simulink model "HeartModelECGPrint"  (R2014a)
settings: Solver=FixedStepDiscrete  StartTime=0.0  StopTime=100  FixedStep=0.01  RelTol=1e-3
values from neighbouring files (symbols this model uses):
  Atr_refrD = 50    [matlab.mat]
  AV_alpha = 150    [matlab.mat]
  AV_anteDMin = 100    [matlab.mat]
  AV_beta = 250    [matlab.mat]
  AV_delta = 10    [matlab.mat]
  AV_k4 = 0.03    [matlab.mat]
  AV_refrDMin = 50    [matlab.mat]
  AV_retroDMin = 100    [matlab.mat]
  AV_tauC = 100    [matlab.mat]
  AV_theta = 10    [matlab.mat]
  AV_tr = 500    [matlab.mat]
  AV_Vr = -90    [matlab.mat]
  AV_Vt = -40    [matlab.mat]
  PM_TAVI = 150    [matlab.mat]
  PM_TLRI = 1000    [matlab.mat]
  PM_TPVAB = 50    [matlab.mat]
  PM_TPVARP = 250    [matlab.mat]
  PM_TURI = 400    [matlab.mat]
  PM_TVRP = 320    [matlab.mat]
  RA_anteD = 75.8904109589    [matlab.mat]
  RA_retroD = 30    [matlab.mat]
  RV_anteD = 50    [matlab.mat]
  RV_retroD = 50    [matlab.mat]
  SA_d = 880.219178082    [matlab.mat]
  SA_dV = 50    [matlab.mat]
  SA_ectopD = 10400    [matlab.mat]
  SA_ectopdV = 50    [matlab.mat]
  SA_noiseD = 1000000    [matlab.mat]
  VRG_d = 3000    [matlab.mat]
  VRG_ectopD = 30450    [matlab.mat]
  VRG_noiseD = 1000000    [matlab.mat]
  Vtr_refrD = 252.054794521    [matlab.mat]
libraries: simulink x4
settings Model: Creator=alexandru  LastModifiedBy=barbot
settings DataIOCC: LimitDataPoints=off  SaveOutput=off  SignalLogging=off  DSMLogging=off  SaveTime=off
settings HardwareCC: TargetBitPerLong=64  TargetBitPerPointer=64  TargetLongLongMode=on  TargetIntDivRoundTo=Zero  TargetEndianess=LittleEndian  TargetWordSize=64  TargetHWDeviceType=MATLAB Host  ProdEqTarget=off
settings RTWCC: SystemTargetFile=rsim.tlc  GenCodeOnly=on  PackageGeneratedCodeAndArtifacts=on  PackageName=idhp_model_heart_realtime  TemplateMakefile=rsim_default_tmf  Description=Rapid Simulation Target  ProcessScript=rsim_make_rtw_hook
settings RSimTargetCC: ERTMultiwordTypeDef=System defined  ERTMultiwordLength=256  EnableShiftOperators=on

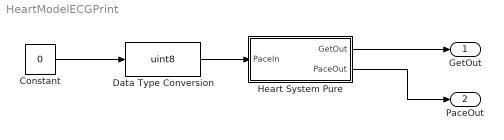
== system HeartModelECGPrint ==
  Constant : Constant  Value=0
  Data Type Conversion : DataTypeConversion  OutDataTypeStr=uint8
  Heart System Pure : Subsystem
  GetOut : Outport
  PaceOut : Outport  Port=2
  wires:
  Data Type Conversion/1 -> Heart System Pure/1(PaceIn)
  Heart System Pure/1(GetOut) -> GetOut/1
  Heart System Pure/2(PaceOut) -> PaceOut/1
  Constant/1 -> Data Type Conversion/1

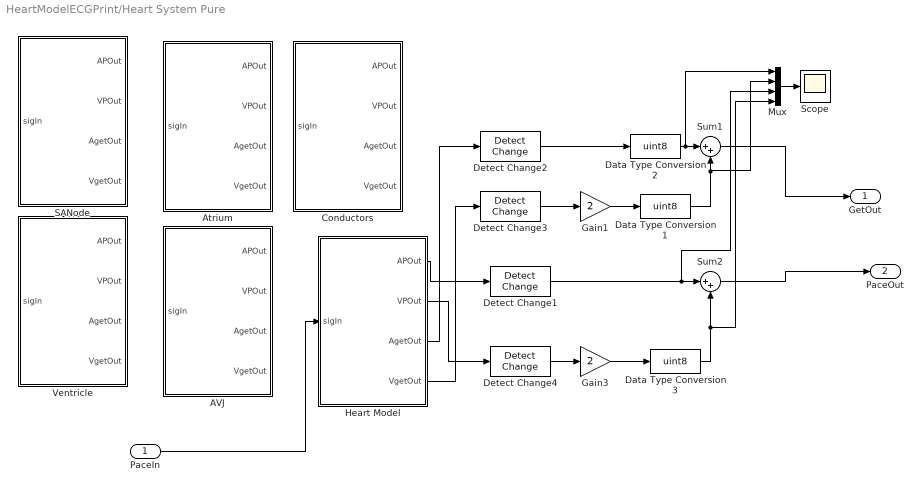
== system HeartModelECGPrint/Heart System Pure ==
  PaceIn : Inport
  AVJ : Stateflow chart  Priority=1  TreatAsAtomicUnit=on
  Atrium : Stateflow chart  Priority=1  TreatAsAtomicUnit=on
  Conductors : Stateflow chart  Priority=1  TreatAsAtomicUnit=on
  Data Type Conversion1 : DataTypeConversion  OutDataTypeStr=uint8
  Data Type Conversion2 : DataTypeConversion  OutDataTypeStr=uint8
  Data Type Conversion3 : DataTypeConversion  OutDataTypeStr=uint8
  Detect Change{1..4} (4 alike) : simulink/Logic and Bit Operations/Detect Change  vinit=0  InputProcessing=Inherited  OutDataTypeStr=uint8
  Gain1 : Gain  Gain=2
  Gain3 : Gain  Gain=2
  Heart Model : Stateflow chart  Priority=1  TreatAsAtomicUnit=on
  Mux : Mux
  SANode : Stateflow chart  Priority=1  TreatAsAtomicUnit=on
  Scope : Scope
  Sum1 : Sum  Inputs=|++
  Sum2 : Sum  Inputs=|++
  Ventricle : Stateflow chart  Priority=1  TreatAsAtomicUnit=on
  GetOut : Outport
  PaceOut : Outport  Port=2
  wires:
  Detect Change3/1 -> Gain1/1
  Gain1/1 -> Data Type Conversion1/1
  Sum1/1 -> GetOut/1
  Data Type Conversion1/1 -> Mux/2, Sum1/2
  Detect Change2/1 -> Data Type Conversion2/1
  Data Type Conversion2/1 -> Mux/1, Sum1/1
  Heart Model/1(APOut) -> Detect Change1/1
  Heart Model/2(VPOut) -> Detect Change4/1
  Detect Change4/1 -> Gain3/1
  Gain3/1 -> Data Type Conversion3/1
  Data Type Conversion3/1 -> Mux/4, Sum2/2
  Detect Change1/1 -> Mux/3, Sum2/1
  Sum2/1 -> PaceOut/1
  PaceIn/1 -> Heart Model/1(sigIn)
  Heart Model/4(VgetOut) -> Detect Change3/1
  Heart Model/3(AgetOut) -> Detect Change2/1
  Mux/1 -> Scope/1

== stateflow chart HeartModelECGPrint/Heart System Pure/SANode ==
  state SANodeEctopic
    state q0
    q0 -> q0 : after(SA_ectopD),
        | !Abeat , {a_dV=SA_ectopdV}
    (default) -> q0
  state SANode
    state Wait4ABeat
    state Wait4ASynch
    Wait4ABeat -> Wait4ASynch [order 2] : after(SA_d),!Abeat,
        | {a_dV=SA_dV}
    (default) -> Wait4ABeat
    Wait4ASynch -> Wait4ABeat : ?NextAtrBeat
    Wait4ABeat -> Wait4ABeat [order 1] : ?NextAtrBeat
  data: Atr_refrD parameter; AV_alpha parameter; AV_anteDMin parameter; AV_beta parameter; AV_delta parameter; AV_k4 parameter; AV_refrDMin parameter; AV_retroDMin parameter; AV_tauC parameter; AV_theta parameter; AV_tr parameter; AV_Vr parameter; AV_Vt parameter; RA_anteD parameter; RA_retroD parameter; RV_anteD parameter; RV_retroD parameter; SA_d parameter; SA_dV parameter; SA_ectopD parameter; SA_ectopdV parameter; SA_noiseD parameter; VRG_d parameter; VRG_ectopD parameter; VRG_noiseD parameter; Vtr_refrD parameter; a_dV local double; avj_tRec local double; sigIn input uint8; clk local double; PM_TAVI parameter; PM_TLRI parameter; PM_TPVAB parameter; PM_TPVARP parameter; PM_TURI parameter; PM_TVRP parameter; data local double
  events: Abeat local FUNCTION_CALL_EVENT; AtrRetroReached local FUNCTION_CALL_EVENT; arg local FUNCTION_CALL_EVENT; retroAVJ local FUNCTION_CALL_EVENT; AVJAnteReached local FUNCTION_CALL_EVENT; NextAtrBeat local FUNCTION_CALL_EVENT; AVJRetroReached local FUNCTION_CALL_EVENT; anteAVJ local FUNCTION_CALL_EVENT; vrg local FUNCTION_CALL_EVENT; VtrAnteReached local FUNCTION_CALL_EVENT; AVJRetroExit local FUNCTION_CALL_EVENT; AVJAnteExit local FUNCTION_CALL_EVENT; NextVtrBeat local FUNCTION_CALL_EVENT; Vbeat local FUNCTION_CALL_EVENT; AP local EITHER_EDGE_EVENT; VP local EITHER_EDGE_EVENT; APOut output EITHER_EDGE_EVENT; VPOut output EITHER_EDGE_EVENT; AS local RISING_EDGE_EVENT; VS local RISING_EDGE_EVENT; Aget local EITHER_EDGE_EVENT; Vget local EITHER_EDGE_EVENT; Aintrinsic local EITHER_EDGE_EVENT; Anoise local EITHER_EDGE_EVENT; Aretro local EITHER_EDGE_EVENT; Vintrinsic local EITHER_EDGE_EVENT; Vnoise local EITHER_EDGE_EVENT; Vante local EITHER_EDGE_EVENT; AgetOut output EITHER_EDGE_EVENT; VgetOut output EITHER_EDGE_EVENT; APElectr local RISING_EDGE_EVENT; VPElectr local EITHER_EDGE_EVENT

== stateflow chart HeartModelECGPrint/Heart System Pure/Heart Model ==
  state Heart
    state SANodeEctopic [parallel]
      settings: executionOrder=10
      state q0
      Heart.SANodeEctopic.q0 -> Heart.SANodeEctopic.q0 : after(SA_ectopD),
          | !Abeat , {a_dV=SA_ectopdV}
      (default) -> Heart.SANodeEctopic.q0
    state RAConductor [parallel]
      settings: executionOrder=3
      state Ante
      state Empty
      state Retro
      Heart.RAConductor.Empty -> Heart.RAConductor.Ante [order 1] : ?arg
      Heart.RAConductor.Ante -> Heart.RAConductor.Empty [order 1] : ?retroAVJ
      (default) -> Heart.RAConductor.Empty
      Heart.RAConductor.Ante -> Heart.RAConductor.Empty [order 2] : after(RA_anteD),
          | !AVJAnteReached
      Heart.RAConductor.Empty -> Heart.RAConductor.Retro [order 2] : ?retroAVJ
      Heart.RAConductor.Retro -> Heart.RAConductor.Empty [order 1] : ?arg
      Heart.RAConductor.Retro -> Heart.RAConductor.Empty [order 2] : after(RA_retroD),
          | !AtrRetroReached
    state AVJOut [parallel]
      settings: executionOrder=1
      state Empty
      state Ante
      state Retro
      Heart.AVJOut.Ante -> Heart.AVJOut.Empty : after(AV_anteDMin+AV_alpha*exp(-avj_tRec/AV_tauC)),
          | !anteAVJ
      (default) -> Heart.AVJOut.Empty
      Heart.AVJOut.Empty -> Heart.AVJOut.Ante [order 1] : ?AVJAnteExit
      Heart.AVJOut.Retro -> Heart.AVJOut.Empty : after(AV_retroDMin+AV_alpha*exp(-avj_tRec/AV_tauC)),
          | !retroAVJ
      Heart.AVJOut.Empty -> Heart.AVJOut.Retro [order 2] : ?AVJRetroExit
    state RVConductor [parallel]
      settings: executionOrder=2
      state Empty
      state Ante
      state Retro
      (default) -> Heart.RVConductor.Empty
      Heart.RVConductor.Empty -> Heart.RVConductor.Ante [order 1] : ?anteAVJ
      Heart.RVConductor.Ante -> Heart.RVConductor.Empty [order 1] : ?vrg
      Heart.RVConductor.Ante -> Heart.RVConductor.Empty [order 2] : after(RV_anteD),
          | !VtrAnteReached
      Heart.RVConductor.Empty -> Heart.RVConductor.Retro [order 2] : ?vrg
      Heart.RVConductor.Retro -> Heart.RVConductor.Empty [order 1] : ?anteAVJ
      Heart.RVConductor.Retro -> Heart.RVConductor.Empty [order 2] : after(RV_retroD),
          | !AVJRetroReached
    state VRGEctopic [parallel]
      settings: executionOrder=8
      state q0
      (default) -> Heart.VRGEctopic.q0
      Heart.VRGEctopic.q0 -> Heart.VRGEctopic.q0 : after(VRG_ectopD), !Vbeat
    state VRG [parallel]
      settings: executionOrder=9
      state Wait4VBeat
      state Wait4VSynch
      (default) -> Wait4VBeat
      Wait4VBeat -> Wait4VSynch [order 2] : after(VRG_d), !Vbeat
      Wait4VSynch -> Wait4VBeat : ?NextVtrBeat
      Wait4VBeat -> Wait4VBeat [order 1] : ?NextVtrBeat
    state SANode [parallel]
      settings: executionOrder=4
      state Wait4ABeat
      state Wait4ASynch
      Wait4ABeat -> Wait4ASynch [order 2] : after(SA_d),!Abeat,
          | {a_dV=SA_dV}
      (default) -> Wait4ABeat
      Wait4ASynch -> Wait4ABeat : ?NextAtrBeat
      Wait4ABeat -> Wait4ABeat [order 1] : ?NextAtrBeat
    state AVJ [parallel]
      settings: executionOrder=7
      state Recovery
      state Ante
      state Refractory
      state Retro
      (default) -> Recovery : {avj_t4=timeToDep(AV_Vr);
          | ctime=0;
          | recoverylast=0;
          | antelast=0;
          | refractorylast=0;}
      Heart.AVJ.Ante -> Heart.AVJ.Refractory : after(avj_t4), !AVJAnteExit, {
          | avj_tRec=avj_tRec+(ctime-antelast);
          | avj_refr_0=initRefrPeriod(avj_tRec);
          | avj_refr=avj_refr_0;
          | refractorylast=ctime;}
      Recovery -> Heart.AVJ.Ante [order 1] : ?AVJAnteReached,{
          | avj_t4 = timeToDep(AV_Vr+ ...
          | (ctime-recoverylast)*AV_k4 + a_dV);
          | avj_tRec=ctime-recoverylast;
          | antelast=ctime;}
      Recovery -> Heart.AVJ.Refractory [order 2] : after(avj_t4), {
          | avj_tRec=avj_t4;
          | avj_refr_0=initRefrPeriod(avj_tRec);
          | avj_refr=avj_refr_0;
          | refractorylast=ctime;}
      Heart.AVJ.Refractory -> Heart.AVJ.Refractory [order 1] : ?AVJAnteReached,{
          | avj_refr=avj_refr-(ctime - refractorylast)+...
          | modulateRefrAnte((ctime - refractorylast),...
          | avj_refr_0,a_dV);
          | refractorylast=ctime;}
      Heart.AVJ.Refractory -> Recovery [order 3] : after(avj_refr), {
          | avj_t4=timeToDep(AV_Vr);
          | recoverylast=ctime;}
      Recovery -> Heart.AVJ.Retro [order 3] : ?AVJRetroReached,{
          | avj_tRec=ctime-recoverylast;
          | avj_refr_0=initRefrPeriod(avj_tRec);
          | avj_refr=avj_refr_0;}
      Heart.AVJ.Retro -> Heart.AVJ.Refractory : !AVJRetroExit, {refractorylast=ctime;}
      Heart.AVJ.Refractory -> Heart.AVJ.Refractory [order 2] : ?AVJRetroReached,{
          | avj_refr=avj_refr-(ctime - refractorylast)+...
          | modulateRefrRetro((ctime - refractorylast),...
          | avj_refr_0);
          | refractorylast=ctime;}
    state Ventricle [parallel]
      settings: executionOrder=5
      state Excitable
      state Refractory
      state VSynch
      state VsenseAnte
      state Vsense
      state GenerateRetroWave
      (default) -> Heart.Ventricle.Refractory
      Heart.Ventricle.Refractory -> Heart.Ventricle.Excitable : after(Vtr_refrD)
      Heart.Ventricle.Excitable -> Vsense [order 3] : ?Vbeat
      Heart.Ventricle.Excitable -> VsenseAnte [order 1] : ?VtrAnteReached
      VSynch -> Heart.Ventricle.Refractory : !NextVtrBeat
      Heart.Ventricle.Excitable -> GenerateRetroWave [order 2] : ?VP, !VPOut
      VsenseAnte -> VSynch : !VgetOut
      GenerateRetroWave -> VSynch : !vrg
      Vsense -> GenerateRetroWave : !VgetOut
    state Atrium [parallel]
      settings: executionOrder=6
      state Excitable
      state Refractory
      state ASynch
      state AsenseRetro
      state Asense
      state GenerateAnteWave
      (default) -> Heart.Atrium.Refractory
      Heart.Atrium.Excitable -> Asense [order 1] : ?Abeat
      Heart.Atrium.Refractory -> Heart.Atrium.Excitable : after(Atr_refrD)
      Heart.Atrium.Excitable -> AsenseRetro [order 3] : ?AtrRetroReached
      ASynch -> Heart.Atrium.Refractory : !NextAtrBeat
      Heart.Atrium.Excitable -> GenerateAnteWave [order 2] : ?AP, !APOut
      AsenseRetro -> ASynch : !AgetOut!
      GenerateAnteWave -> ASynch : !arg
      Asense -> GenerateAnteWave : !AgetOut!
  (default) -> Heart
  data: avj_refr local double; avj_t4 local double; avj_refr_0 local double; ctime local double; recoverylast local double; antelast local double; refractorylast local double; Atr_refrD parameter; AV_alpha parameter; AV_anteDMin parameter; AV_beta parameter; AV_delta parameter; AV_k4 parameter; AV_refrDMin parameter; AV_retroDMin parameter; AV_tauC parameter; AV_theta parameter; AV_tr parameter; AV_Vr parameter; AV_Vt parameter; RA_anteD parameter; RA_retroD parameter; RV_anteD parameter; RV_retroD parameter; SA_d parameter; SA_dV parameter; SA_ectopD parameter; SA_ectopdV parameter; SA_noiseD parameter; VRG_d parameter; VRG_ectopD parameter; VRG_noiseD parameter; Vtr_refrD parameter; a_dV local double; avj_tRec local double; sigIn input uint8; clk local double; PM_TAVI parameter; PM_TLRI parameter; PM_TPVAB parameter; PM_TPVARP parameter; PM_TURI parameter; PM_TVRP parameter; data local double
  events: Abeat local FUNCTION_CALL_EVENT; AtrRetroReached local FUNCTION_CALL_EVENT; arg local FUNCTION_CALL_EVENT; retroAVJ local FUNCTION_CALL_EVENT; AVJAnteReached local FUNCTION_CALL_EVENT; NextAtrBeat local FUNCTION_CALL_EVENT; AVJRetroReached local FUNCTION_CALL_EVENT; anteAVJ local FUNCTION_CALL_EVENT; vrg local FUNCTION_CALL_EVENT; VtrAnteReached local FUNCTION_CALL_EVENT; AVJRetroExit local FUNCTION_CALL_EVENT; AVJAnteExit local FUNCTION_CALL_EVENT; NextVtrBeat local FUNCTION_CALL_EVENT; Vbeat local FUNCTION_CALL_EVENT; AP local EITHER_EDGE_EVENT; VP local EITHER_EDGE_EVENT; APOut output EITHER_EDGE_EVENT; VPOut output EITHER_EDGE_EVENT; AS local RISING_EDGE_EVENT; VS local RISING_EDGE_EVENT; Aget local EITHER_EDGE_EVENT; Vget local EITHER_EDGE_EVENT; Aintrinsic local EITHER_EDGE_EVENT; Anoise local EITHER_EDGE_EVENT; Aretro local EITHER_EDGE_EVENT; Vintrinsic local EITHER_EDGE_EVENT; Vnoise local EITHER_EDGE_EVENT; Vante local EITHER_EDGE_EVENT; AgetOut output EITHER_EDGE_EVENT; VgetOut output EITHER_EDGE_EVENT; APElectr local RISING_EDGE_EVENT; VPElectr local EITHER_EDGE_EVENT

== stateflow chart HeartModelECGPrint/Heart System Pure/Atrium ==
  state Atrium
    state Excitable
    state Refractory
    state ASynch
    state AsenseRetro
    state Asense
    state GenerateAnteWave
    (default) -> Refractory
    Excitable -> Asense [order 1] : ?Abeat
    Refractory -> Excitable : after(Atr_refrD)
    Excitable -> AsenseRetro [order 3] : ?AtrRetroReached
    ASynch -> Refractory : !NextAtrBeat
    Excitable -> GenerateAnteWave [order 2] : ?AP, !APOut
    AsenseRetro -> ASynch : !AgetOut!
    GenerateAnteWave -> ASynch : !arg
    Asense -> GenerateAnteWave : !AgetOut!
  data: Atr_refrD parameter; AV_alpha parameter; AV_anteDMin parameter; AV_beta parameter; AV_delta parameter; AV_k4 parameter; AV_refrDMin parameter; AV_retroDMin parameter; AV_tauC parameter; AV_theta parameter; AV_tr parameter; AV_Vr parameter; AV_Vt parameter; RA_anteD parameter; RA_retroD parameter; RV_anteD parameter; RV_retroD parameter; SA_d parameter; SA_dV parameter; SA_ectopD parameter; SA_ectopdV parameter; SA_noiseD parameter; VRG_d parameter; VRG_ectopD parameter; VRG_noiseD parameter; Vtr_refrD parameter; a_dV local double; avj_tRec local double; sigIn input uint8; clk local double; PM_TAVI parameter; PM_TLRI parameter; PM_TPVAB parameter; PM_TPVARP parameter; PM_TURI parameter; PM_TVRP parameter; data local double
  events: Abeat local FUNCTION_CALL_EVENT; AtrRetroReached local FUNCTION_CALL_EVENT; arg local FUNCTION_CALL_EVENT; retroAVJ local FUNCTION_CALL_EVENT; AVJAnteReached local FUNCTION_CALL_EVENT; NextAtrBeat local FUNCTION_CALL_EVENT; AVJRetroReached local FUNCTION_CALL_EVENT; anteAVJ local FUNCTION_CALL_EVENT; vrg local FUNCTION_CALL_EVENT; VtrAnteReached local FUNCTION_CALL_EVENT; AVJRetroExit local FUNCTION_CALL_EVENT; AVJAnteExit local FUNCTION_CALL_EVENT; NextVtrBeat local FUNCTION_CALL_EVENT; Vbeat local FUNCTION_CALL_EVENT; AP local EITHER_EDGE_EVENT; VP local EITHER_EDGE_EVENT; APOut output EITHER_EDGE_EVENT; VPOut output EITHER_EDGE_EVENT; AS local RISING_EDGE_EVENT; VS local RISING_EDGE_EVENT; Aget local EITHER_EDGE_EVENT; Vget local EITHER_EDGE_EVENT; Aintrinsic local EITHER_EDGE_EVENT; Anoise local EITHER_EDGE_EVENT; Aretro local EITHER_EDGE_EVENT; Vintrinsic local EITHER_EDGE_EVENT; Vnoise local EITHER_EDGE_EVENT; Vante local EITHER_EDGE_EVENT; AgetOut output EITHER_EDGE_EVENT; VgetOut output EITHER_EDGE_EVENT; APElectr local RISING_EDGE_EVENT; VPElectr local EITHER_EDGE_EVENT

== stateflow chart HeartModelECGPrint/Heart System Pure/Conductors ==
  state RAConductor
    state Ante
    state Empty
    state Retro
    RAConductor.Empty -> RAConductor.Ante [order 1] : ?arg
    RAConductor.Ante -> RAConductor.Empty [order 1] : ?retroAVJ
    (default) -> RAConductor.Empty
    RAConductor.Ante -> RAConductor.Empty [order 2] : after(RA_anteD),
        | !AVJAnteReached
    RAConductor.Empty -> RAConductor.Retro [order 2] : ?retroAVJ
    RAConductor.Retro -> RAConductor.Empty [order 1] : ?arg
    RAConductor.Retro -> RAConductor.Empty [order 2] : after(RA_retroD),
        | !AtrRetroReached
  state RVConductor
    state Empty
    state Ante
    state Retro
    (default) -> RVConductor.Empty
    RVConductor.Empty -> RVConductor.Ante [order 1] : ?anteAVJ
    RVConductor.Ante -> RVConductor.Empty [order 1] : ?vrg
    RVConductor.Ante -> RVConductor.Empty [order 2] : after(RV_anteD),
        | !VtrAnteReached
    RVConductor.Empty -> RVConductor.Retro [order 2] : ?vrg
    RVConductor.Retro -> RVConductor.Empty [order 1] : ?anteAVJ
    RVConductor.Retro -> RVConductor.Empty [order 2] : after(RV_retroD),
        | !AVJRetroReached
  data: Atr_refrD parameter; AV_alpha parameter; AV_anteDMin parameter; AV_beta parameter; AV_delta parameter; AV_k4 parameter; AV_refrDMin parameter; AV_retroDMin parameter; AV_tauC parameter; AV_theta parameter; AV_tr parameter; AV_Vr parameter; AV_Vt parameter; RA_anteD parameter; RA_retroD parameter; RV_anteD parameter; RV_retroD parameter; SA_d parameter; SA_dV parameter; SA_ectopD parameter; SA_ectopdV parameter; SA_noiseD parameter; VRG_d parameter; VRG_ectopD parameter; VRG_noiseD parameter; Vtr_refrD parameter; a_dV local double; avj_tRec local double; sigIn input uint8; clk local double; PM_TAVI parameter; PM_TLRI parameter; PM_TPVAB parameter; PM_TPVARP parameter; PM_TURI parameter; PM_TVRP parameter; data local double
  events: Abeat local FUNCTION_CALL_EVENT; AtrRetroReached local FUNCTION_CALL_EVENT; arg local FUNCTION_CALL_EVENT; retroAVJ local FUNCTION_CALL_EVENT; AVJAnteReached local FUNCTION_CALL_EVENT; NextAtrBeat local FUNCTION_CALL_EVENT; AVJRetroReached local FUNCTION_CALL_EVENT; anteAVJ local FUNCTION_CALL_EVENT; vrg local FUNCTION_CALL_EVENT; VtrAnteReached local FUNCTION_CALL_EVENT; AVJRetroExit local FUNCTION_CALL_EVENT; AVJAnteExit local FUNCTION_CALL_EVENT; NextVtrBeat local FUNCTION_CALL_EVENT; Vbeat local FUNCTION_CALL_EVENT; AP local EITHER_EDGE_EVENT; VP local EITHER_EDGE_EVENT; APOut output EITHER_EDGE_EVENT; VPOut output EITHER_EDGE_EVENT; AS local RISING_EDGE_EVENT; VS local RISING_EDGE_EVENT; Aget local EITHER_EDGE_EVENT; Vget local EITHER_EDGE_EVENT; Aintrinsic local EITHER_EDGE_EVENT; Anoise local EITHER_EDGE_EVENT; Aretro local EITHER_EDGE_EVENT; Vintrinsic local EITHER_EDGE_EVENT; Vnoise local EITHER_EDGE_EVENT; Vante local EITHER_EDGE_EVENT; AgetOut output EITHER_EDGE_EVENT; VgetOut output EITHER_EDGE_EVENT; APElectr local RISING_EDGE_EVENT; VPElectr local EITHER_EDGE_EVENT

== stateflow chart HeartModelECGPrint/Heart System Pure/Ventricle ==
  state VRGEctopic
    state q0
    (default) -> q0
    q0 -> q0 : after(VRG_ectopD), !Vbeat
  state Ventricle
    state Excitable
    state Refractory
    state VSynch
    state VsenseAnte
    state Vsense
    state GenerateRetroWave
    (default) -> Refractory
    Refractory -> Excitable : after(Vtr_refrD)
    Excitable -> Vsense [order 3] : ?Vbeat
    Excitable -> VsenseAnte [order 1] : ?VtrAnteReached
    VSynch -> Refractory : !NextVtrBeat
    Excitable -> GenerateRetroWave [order 2] : ?VP, !VPOut
    VsenseAnte -> VSynch : !VgetOut
    GenerateRetroWave -> VSynch : !vrg
    Vsense -> GenerateRetroWave : !VgetOut
  state VRG
    state Wait4VBeat
    state Wait4VSynch
    (default) -> Wait4VBeat
    Wait4VBeat -> Wait4VSynch [order 2] : after(VRG_d), !Vbeat
    Wait4VSynch -> Wait4VBeat : ?NextVtrBeat
    Wait4VBeat -> Wait4VBeat [order 1] : ?NextVtrBeat
  data: Atr_refrD parameter; AV_alpha parameter; AV_anteDMin parameter; AV_beta parameter; AV_delta parameter; AV_k4 parameter; AV_refrDMin parameter; AV_retroDMin parameter; AV_tauC parameter; AV_theta parameter; AV_tr parameter; AV_Vr parameter; AV_Vt parameter; RA_anteD parameter; RA_retroD parameter; RV_anteD parameter; RV_retroD parameter; SA_d parameter; SA_dV parameter; SA_ectopD parameter; SA_ectopdV parameter; SA_noiseD parameter; VRG_d parameter; VRG_ectopD parameter; VRG_noiseD parameter; Vtr_refrD parameter; a_dV local double; avj_tRec local double; sigIn input uint8; clk local double; PM_TAVI parameter; PM_TLRI parameter; PM_TPVAB parameter; PM_TPVARP parameter; PM_TURI parameter; PM_TVRP parameter; data local double
  events: Abeat local FUNCTION_CALL_EVENT; AtrRetroReached local FUNCTION_CALL_EVENT; arg local FUNCTION_CALL_EVENT; retroAVJ local FUNCTION_CALL_EVENT; AVJAnteReached local FUNCTION_CALL_EVENT; NextAtrBeat local FUNCTION_CALL_EVENT; AVJRetroReached local FUNCTION_CALL_EVENT; anteAVJ local FUNCTION_CALL_EVENT; vrg local FUNCTION_CALL_EVENT; VtrAnteReached local FUNCTION_CALL_EVENT; AVJRetroExit local FUNCTION_CALL_EVENT; AVJAnteExit local FUNCTION_CALL_EVENT; NextVtrBeat local FUNCTION_CALL_EVENT; Vbeat local FUNCTION_CALL_EVENT; AP local EITHER_EDGE_EVENT; VP local EITHER_EDGE_EVENT; APOut output EITHER_EDGE_EVENT; VPOut output EITHER_EDGE_EVENT; AS local RISING_EDGE_EVENT; VS local RISING_EDGE_EVENT; Aget local EITHER_EDGE_EVENT; Vget local EITHER_EDGE_EVENT; Aintrinsic local EITHER_EDGE_EVENT; Anoise local EITHER_EDGE_EVENT; Aretro local EITHER_EDGE_EVENT; Vintrinsic local EITHER_EDGE_EVENT; Vnoise local EITHER_EDGE_EVENT; Vante local EITHER_EDGE_EVENT; AgetOut output EITHER_EDGE_EVENT; VgetOut output EITHER_EDGE_EVENT; APElectr local RISING_EDGE_EVENT; VPElectr local EITHER_EDGE_EVENT

== stateflow chart HeartModelECGPrint/Heart System Pure/AVJ ==
  state AVJOut
    state Empty
    state Ante
    state Retro
    AVJOut.Ante -> Empty : after(AV_anteDMin+AV_alpha*exp(-avj_tRec/AV_tauC)),
        | !anteAVJ
    (default) -> Empty
    Empty -> AVJOut.Ante [order 1] : ?AVJAnteExit
    AVJOut.Retro -> Empty : after(AV_retroDMin+AV_alpha*exp(-avj_tRec/AV_tauC)),
        | !retroAVJ
    Empty -> AVJOut.Retro [order 2] : ?AVJRetroExit
  state AVJ
    state Recovery
    state Ante
    state Refractory
    state Retro
    (default) -> Recovery : {avj_t4=timeToDep(AV_Vr);
        | ctime=0;
        | recoverylast=0;
        | antelast=0;
        | refractorylast=0;}
    AVJ.Ante -> Refractory : after(avj_t4), !AVJAnteExit, {
        | avj_tRec=avj_tRec+(ctime-antelast);
        | avj_refr_0=initRefrPeriod(avj_tRec);
        | avj_refr=avj_refr_0;
        | refractorylast=ctime;}
    Recovery -> AVJ.Ante [order 1] : ?AVJAnteReached,{
        | avj_t4 = timeToDep(AV_Vr+ ...
        | (ctime-recoverylast)*AV_k4 + a_dV);
        | avj_tRec=ctime-recoverylast;
        | antelast=ctime;}
    Recovery -> Refractory [order 2] : after(avj_t4), {
        | avj_tRec=avj_t4;
        | avj_refr_0=initRefrPeriod(avj_tRec);
        | avj_refr=avj_refr_0;
        | refractorylast=ctime;}
    Refractory -> Refractory [order 1] : ?AVJAnteReached,{
        | avj_refr=avj_refr-(ctime - refractorylast)+...
        | modulateRefrAnte((ctime - refractorylast),...
        | avj_refr_0,a_dV);
        | refractorylast=ctime;}
    Refractory -> Recovery [order 3] : after(avj_refr), {
        | avj_t4=timeToDep(AV_Vr);
        | recoverylast=ctime;}
    Recovery -> AVJ.Retro [order 3] : ?AVJRetroReached,{
        | avj_tRec=ctime-recoverylast;
        | avj_refr_0=initRefrPeriod(avj_tRec);
        | avj_refr=avj_refr_0;}
    AVJ.Retro -> Refractory : !AVJRetroExit, {refractorylast=ctime;}
    Refractory -> Refractory [order 2] : ?AVJRetroReached,{
        | avj_refr=avj_refr-(ctime - refractorylast)+...
        | modulateRefrRetro((ctime - refractorylast),...
        | avj_refr_0);
        | refractorylast=ctime;}
  data: avj_refr local double; avj_t4 local double; avj_refr_0 local double; ctime local double; recoverylast local double; antelast local double; refractorylast local double; Atr_refrD parameter; AV_alpha parameter; AV_anteDMin parameter; AV_beta parameter; AV_delta parameter; AV_k4 parameter; AV_refrDMin parameter; AV_retroDMin parameter; AV_tauC parameter; AV_theta parameter; AV_tr parameter; AV_Vr parameter; AV_Vt parameter; RA_anteD parameter; RA_retroD parameter; RV_anteD parameter; RV_retroD parameter; SA_d parameter; SA_dV parameter; SA_ectopD parameter; SA_ectopdV parameter; SA_noiseD parameter; VRG_d parameter; VRG_ectopD parameter; VRG_noiseD parameter; Vtr_refrD parameter; a_dV local double; avj_tRec local double; sigIn input uint8; clk local double; PM_TAVI parameter; PM_TLRI parameter; PM_TPVAB parameter; PM_TPVARP parameter; PM_TURI parameter; PM_TVRP parameter; data local double
  events: Abeat local FUNCTION_CALL_EVENT; AtrRetroReached local FUNCTION_CALL_EVENT; arg local FUNCTION_CALL_EVENT; retroAVJ local FUNCTION_CALL_EVENT; AVJAnteReached local FUNCTION_CALL_EVENT; NextAtrBeat local FUNCTION_CALL_EVENT; AVJRetroReached local FUNCTION_CALL_EVENT; anteAVJ local FUNCTION_CALL_EVENT; vrg local FUNCTION_CALL_EVENT; VtrAnteReached local FUNCTION_CALL_EVENT; AVJRetroExit local FUNCTION_CALL_EVENT; AVJAnteExit local FUNCTION_CALL_EVENT; NextVtrBeat local FUNCTION_CALL_EVENT; Vbeat local FUNCTION_CALL_EVENT; AP local EITHER_EDGE_EVENT; VP local EITHER_EDGE_EVENT; APOut output EITHER_EDGE_EVENT; VPOut output EITHER_EDGE_EVENT; AS local RISING_EDGE_EVENT; VS local RISING_EDGE_EVENT; Aget local EITHER_EDGE_EVENT; Vget local EITHER_EDGE_EVENT; Aintrinsic local EITHER_EDGE_EVENT; Anoise local EITHER_EDGE_EVENT; Aretro local EITHER_EDGE_EVENT; Vintrinsic local EITHER_EDGE_EVENT; Vnoise local EITHER_EDGE_EVENT; Vante local EITHER_EDGE_EVENT; AgetOut output EITHER_EDGE_EVENT; VgetOut output EITHER_EDGE_EVENT; APElectr local RISING_EDGE_EVENT; VPElectr local EITHER_EDGE_EVENT
